simulink model "kalman"  (R2023a)
settings: Solver=VariableStepAuto  StartTime=0.0  StopTime=0.5  RelTol=1e-3
values from neighbouring files (symbols this model uses):
  B_tilda = [sysdis.B(1) Bw_bar(1,1) Bw_bar(1,2); sysdis.B(2) Bw_bar(2,1) Bw_bar(2,2)]    [motor.m]
  D_tilda = [0 0 0 ; 0 0 0]    [motor.m]
  N = 10    [motor.m]    (also in motor_mpc.m = 3; mpc_unconstrained.m)
  Q_LQ = eye(2)    [motor.m]
  R_LQ = 1    [motor.m]
  sysdis = c2d(sys,Ts)    [motor.m]
  Ts = 0.001    [parameters.m]
  u_max = 12    [constraints.m]
  u_min = 0    [constraints.m]
  uBar = -(A(1,1)*(-A(2,2)*nref/A(2,1)) + A(1,2)*nref)*L    [motor.m]
  w = [1 1]'    [parameters.m]
  x0 = [0.2 70.3]'    [motor.m]
  x_max = [x1_max;x2_max]    [constraints.m]
  x_min = [x1_min;x2_min]    [constraints.m]
  yref = [iref nref]'    [motor.m]
undefined symbols (not defined in the file or in its folder): Discrete, motor_mpc, Sd, Time
libraries: ctrlSharedLib x1, simulink x1
settings Model: Creator=teora  LastModifiedBy=teora

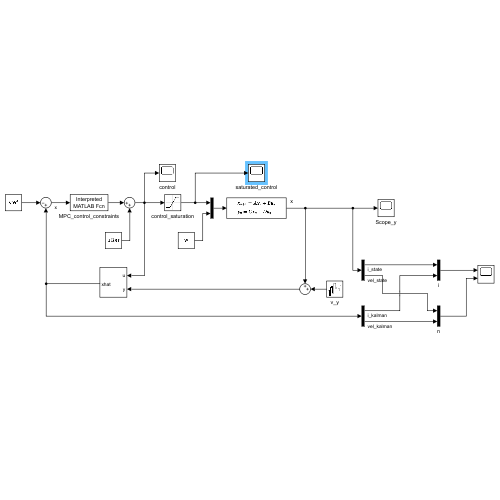
[thumbnail: Simulink's stored preview of the top-level diagram]
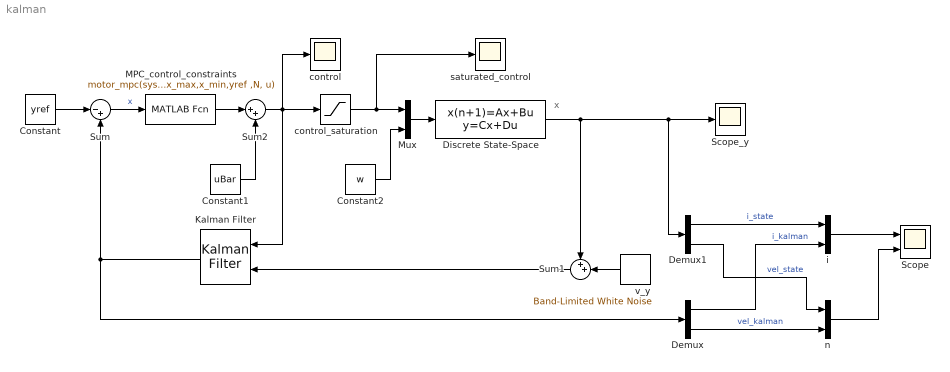
== system kalman ==
  note: x
  Constant : Constant  Value=yref
  Constant1 : Constant  Value=uBar
  Constant2 : Constant  Value=w  SampleTime=Ts
  Demux : Demux  Outputs=2
  Demux1 : Demux  Outputs=2
  Discrete State-Space : DiscreteStateSpace  A=sysdis.A  B=B_tilda  C=sysdis.C  D=D_tilda  InitialCondition=x0  SampleTime=Ts
  Kalman Filter : ctrlSharedLib/Kalman Filter  TimeDomain=Discrete-Time  UseCurrentEstimator=on  ModelSource=Individual A, B, C, D matrices  ModelSourceVariable=ss(0.95,1,1,0,1)  A=sysdis.A  B=sysdis.B  C=sysdis.C  D=sysdis.D  NumberOfStates=1  NumberOfInputs=1  NumberOfOutputs=1  InitialEstimateSource=Dialog  X0=x0  P0=10  UseK=off  UseGH=off  NumberOfProcessNoiseInputs=1  G=1  TimeInvariantG=on  H=0  TimeInvariantH=on  Q=10000  TimeInvariantQ=on  R=1  TimeInvariantR=on  N=0  TimeInvariantN=on  AddInputPort=on  AddEnablePort=off  OutputEstimatedY=off  OutputP=off  Ts=Ts
  MPC_control_constraints : MATLABFcn  MATLABFcn=motor_mpc(sysdis.A, sysdis.B, Q_LQ, R_LQ, Sd, u_max, u_min, x_max,x_min,yref ,N, u)  OutputDimensions=1
  Mux : Mux  Inputs=2
  Scope : Scope  NumInputPorts=2
  Scope_y : Scope
  Sum : Sum  Inputs=|-+
  Sum1 : Sum  Inputs=++|
  Sum2 : Sum  Inputs=|++
  control : Scope
  control_saturation : Saturate  UpperLimit=u_max  LowerLimit=u_min
  i : Mux  Inputs=2
  n : Mux  Inputs=2
  saturated_control : Scope
  v_y : simulink/Sources/Band-Limited White Noise  Cov=[0.0001]  Ts=Ts  seed=[23341]
  wires:
  control_saturation/1 -> Mux/1, saturated_control/1
  Constant/1 -> Sum/1
  Kalman Filter/1 -> Sum/2, Demux/1
  Discrete State-Space/1 -> Scope_y/1, Demux1/1, Sum1/1
  Demux/2 -> n/2  "vel_kalman"
  Demux1/1 -> i/1  "i_state"
  Constant2/1 -> Mux/2
  Mux/1 -> Discrete State-Space/1
  n/1 -> Scope/2
  MPC_control_constraints/1 -> Sum2/1
  i/1 -> Scope/1
  Constant1/1 -> Sum2/2
  Sum2/1 -> control/1, control_saturation/1, Kalman Filter/1
  Sum/1 -> MPC_control_constraints/1  "x"
  Demux/1 -> i/2  "i_kalman"
  Demux1/2 -> n/1  "vel_state"
  v_y/1 -> Sum1/2
  Sum1/1 -> Kalman Filter/2
